simulink model "cx06_MA"  (Simulink 7.5)
settings: Solver=FixedStepDiscrete  StartTime=0.0  StopTime=10.0  RelTol=1e-3
undefined symbols (not defined in the file or in its folder): DiscIntNeverNeededParam, ECU555, int, motohawk_build_version, motohawk_trunc_name, motohawk_vardec_path
libraries: MotoHawk_lib x811, simulink x43, simulink_need_slupdate x1
(part 3 of 10)

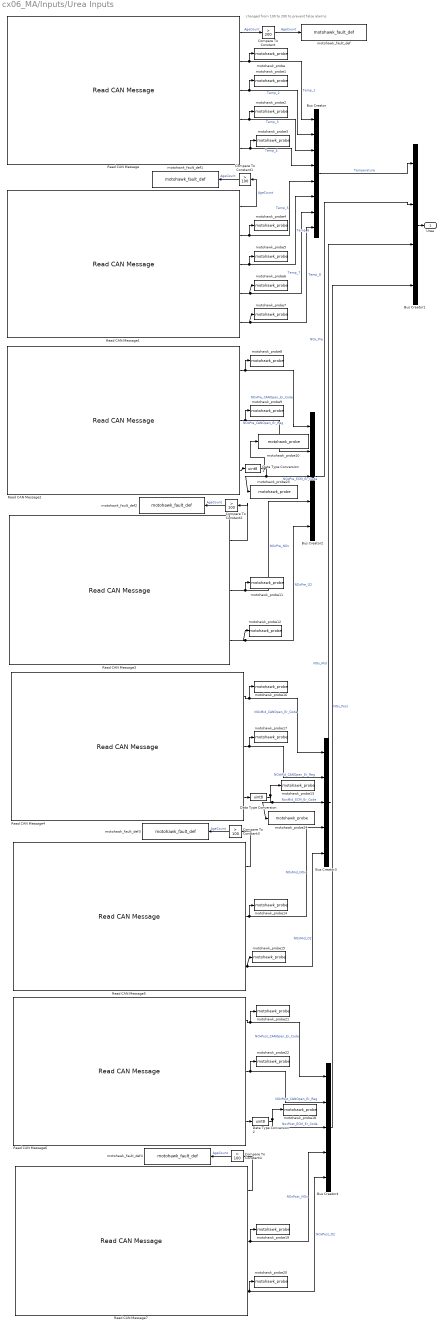
== system cx06_MA/Inputs/Urea Inputs ==
  note: changed from 100 to 200 to prevent false alarms
  Bus Creator : BusCreator  Inputs=8
  Bus Creator1 : BusCreator
  Bus Creator2 : BusCreator  Inputs=5
  Bus Creator3 : BusCreator  Inputs=5
  Bus Creator4 : BusCreator  Inputs=5
  Compare To Constant : simulink/Logic and Bit Operations/Compare To Constant  SystemSampleTime=-1  relop=>  const=200  LogicOutDataTypeMode=boolean  ZeroCross=off
  Compare To Constant{1..4} (4 alike) : simulink/Logic and Bit Operations/Compare To Constant  SystemSampleTime=-1  relop=>  const=100  LogicOutDataTypeMode=boolean  ZeroCross=off
  Data Type Conversion : DataTypeConversion  OutDataTypeMode=uint8  OutDataType=sfix(16)  OutScaling=2^0  OutDataTypeStr=uint8
  Data Type Conversion1 : DataTypeConversion  OutDataTypeMode=uint8  OutDataType=sfix(16)  OutScaling=2^0  OutDataTypeStr=uint8
  Data Type Conversion2 : DataTypeConversion  OutDataTypeMode=uint8  OutDataType=sfix(16)  OutScaling=2^0  OutDataTypeStr=uint8
  Read CAN Message : MotoHawk_lib/CAN Blocks/Read CAN Message  nam=['CAN_' num2str(1)]  bus=-2  msg=CANRx_Temp_1A4  queue=1  slot=''  valid=off  stale=on  labelwires=on
  Read CAN Message1 : MotoHawk_lib/CAN Blocks/Read CAN Message  nam=['CAN_' num2str(1)]  bus=-2  msg=CANRx_Temp_1A5  queue=1  slot=''  valid=off  stale=on  labelwires=on
  Read CAN Message2 : MotoHawk_lib/CAN Blocks/Read CAN Message  nam=['CAN_' num2str(1)]  bus=-2  msg=CANRx_NOx_A3  queue=1  slot=''  valid=off  stale=off  labelwires=off
  Read CAN Message3 : MotoHawk_lib/CAN Blocks/Read CAN Message  nam=['CAN_' num2str(1)]  bus=-2  msg=CANRx_NOx_1A3  queue=1  slot=''  valid=off  stale=on  labelwires=off
  Read CAN Message4 : MotoHawk_lib/CAN Blocks/Read CAN Message  nam=['CAN_' num2str(1)]  bus=-2  msg=CANRx_NOx_A1  queue=1  slot=''  valid=off  stale=off  labelwires=off
  Read CAN Message5 : MotoHawk_lib/CAN Blocks/Read CAN Message  nam=['CAN_' num2str(1)]  bus=-2  msg=CANRx_NOx_1A1  queue=1  slot=''  valid=off  stale=on  labelwires=off
  Read CAN Message6 : MotoHawk_lib/CAN Blocks/Read CAN Message  nam=['CAN_' num2str(1)]  bus=-2  msg=CANRx_NOx_A2  queue=1  slot=''  valid=off  stale=off  labelwires=off
  Read CAN Message7 : MotoHawk_lib/CAN Blocks/Read CAN Message  nam=['CAN_' num2str(1)]  bus=-2  msg=CANRx_NOx_1A2  queue=1  slot=''  valid=off  stale=on  labelwires=off
  motohawk_fault_def : MotoHawk_lib/Fault Management Blocks/motohawk_fault_def  nam='Temp1A4'  mode=Enabled - Persistent  id=[]  x=10  y=11  input_suspected=on  indeterminate=off  increment_xy=on  downsample_count=1  ovr_cals=on  ovr_actions=on  show_actions=on  action1_name='Urea_Inject'  action1_cond=Active  action2_name=''  action2_cond=(None)  action3_name=''  action3_cond=(None)  action4_name=''  action4_cond=(None)
  motohawk_fault_def1 : MotoHawk_lib/Fault Management Blocks/motohawk_fault_def  nam='Temp1A5'  mode=Enabled - Persistent  id=[]  x=10  y=11  input_suspected=on  indeterminate=off  increment_xy=on  downsample_count=1  ovr_cals=on  ovr_actions=on  show_actions=on  action1_name=''  action1_cond=(None)  action2_name=''  action2_cond=(None)  action3_name=''  action3_cond=(None)  action4_name=''  action4_cond=(None)
  motohawk_fault_def2 : MotoHawk_lib/Fault Management Blocks/motohawk_fault_def  nam='NOxPre_CAN'  mode=Enabled - Persistent  id=[]  x=10  y=11  input_suspected=on  indeterminate=off  increment_xy=on  downsample_count=1  ovr_cals=on  ovr_actions=on  show_actions=on  action1_name='Urea_Inject'  action1_cond=Active  action2_name=''  action2_cond=(None)  action3_name=''  action3_cond=(None)  action4_name=''  action4_cond=(None)
  motohawk_fault_def3 : MotoHawk_lib/Fault Management Blocks/motohawk_fault_def  nam='NOxMid_CAN'  mode=Enabled - Persistent  id=[]  x=10  y=11  input_suspected=on  indeterminate=off  increment_xy=on  downsample_count=1  ovr_cals=on  ovr_actions=on  show_actions=on  action1_name=''  action1_cond=(None)  action2_name=''  action2_cond=(None)  action3_name=''  action3_cond=(None)  action4_name=''  action4_cond=(None)
  motohawk_fault_def4 : MotoHawk_lib/Fault Management Blocks/motohawk_fault_def  nam='NOxPost_CAN'  mode=Enabled - Persistent  id=[]  x=10  y=11  input_suspected=on  indeterminate=off  increment_xy=on  downsample_count=1  ovr_cals=on  ovr_actions=on  show_actions=on  action1_name=''  action1_cond=(None)  action2_name=''  action2_cond=(None)  action3_name=''  action3_cond=(None)  action4_name=''  action4_cond=(None)
  motohawk_probe{,1..9,11..12,14..17,19..22} (20 alike) : MotoHawk_lib/Calibration & Probing Blocks/motohawk_probe  nam='Probe'  show_more=on  name_source=Use Input Wire Name  read_level=1  view_as=Number  enum_struct={'Disabled', 'Enabled'}  vector_style=Wide Row  use_help_units=off  help=''  units=''  use_header_enum=off  row_header_enum={}  col_header_enum={}  use_precision=off  precision=''  gain=1  offset=0  exp=1  use_mototune_group=off  mototune_group=motohawk_vardec_path(gcb)
  motohawk_probe10 : MotoHawk_lib/Calibration & Probing Blocks/motohawk_probe  nam='Probe'  show_more=on  name_source=Use Input Wire Name  read_level=1  view_as=Enumeration  enum_struct=struct('name', {'All OK', '16b ADC failed to init', '+Vsw shorted', 'Sensor Turned Off', 'HTR Open', 'HTR Shorted', '1wire bus Shorted', 'No 1wire bus', 'CRC16 Error', 'Invalid 1wire par', '+Vsw < 9 for 7s', '+Vsw > 30V', 'VS > 1.5/1.6V', 'RVS > 280/300', 'VHerr > 0.5V', 'VP1+ > 6V', 'VP2+ < 2V', 'VP2 out range', '.25V>VS+>.75V', 'UserData Corrupt', 'Invld SW State', 'CAN overrun', 'CAN passive', 'CAN heartbeat', 'CAN recover bus off', 'CAN TxID col', 'Serial Overrun'}, 'value', {0, 17, 18, 19, 20, 21, 33, 34, 35, 36, 49, 50, 65, 81, 82, 97, 98, 99, 100, 101, 161, 177, 178, 179, 180, 181, 182})  vector_style=Wide Row  use_help_units=off  help=''  units=''  use_header_enum=off  row_header_enum={}  col_header_enum={}  use_precision=off  precision=''  gain=1  offset=0  exp=1  use_mototune_group=off  mototune_group=motohawk_vardec_path(gcb)
  motohawk_probe13 : MotoHawk_lib/Calibration & Probing Blocks/motohawk_probe  nam='Probe'  show_more=on  name_source=Use Input Wire Name  read_level=1  view_as=Enumeration  enum_struct=struct('name', {'All OK', '16b ADC failed to init', '+Vsw shorted', 'Sensor Turned Off', 'HTR Open', 'HTR Shorted', '1wire bus Shorted', 'No 1wire bus', 'CRC16 Error', 'Invalid 1wire par', '+Vsw < 9 for 7s', '+Vsw > 30V', 'VS > 1.5/1.6V', 'RVS > 280/300', 'VHerr > 0.5V', 'VP1+ > 6V', 'VP2+ < 2V', 'VP2 out range', '.25V>VS+>.75V', 'UserData Corrupt', 'Invld SW State', 'CAN overrun', 'CAN passive', 'CAN heartbeat', 'CAN recover bus off', 'CAN TxID col', 'Serial Overrun'}, 'value', {0, 17, 18, 19, 20, 21, 33, 34, 35, 36, 49, 50, 65, 81, 82, 97, 98, 99, 100, 101, 161, 177, 178, 179, 180, 181, 182})  vector_style=Wide Row  use_help_units=off  help=''  units=''  use_header_enum=off  row_header_enum={}  col_header_enum={}  use_precision=off  precision=''  gain=1  offset=0  exp=1  use_mototune_group=off  mototune_group=motohawk_vardec_path(gcb)
  motohawk_probe18 : MotoHawk_lib/Calibration & Probing Blocks/motohawk_probe  nam='Probe'  show_more=on  name_source=Use Input Wire Name  read_level=1  view_as=Enumeration  enum_struct=struct('name', {'All OK', '16b ADC failed to init', '+Vsw shorted', 'Sensor Turned Off', 'HTR Open', 'HTR Shorted', '1wire bus Shorted', 'No 1wire bus', 'CRC16 Error', 'Invalid 1wire par', '+Vsw < 9 for 7s', '+Vsw > 30V', 'VS > 1.5/1.6V', 'RVS > 280/300', 'VHerr > 0.5V', 'VP1+ > 6V', 'VP2+ < 2V', 'VP2 out range', '.25V>VS+>.75V', 'UserData Corrupt', 'Invld SW State', 'CAN overrun', 'CAN passive', 'CAN heartbeat', 'CAN recover bus off', 'CAN TxID col', 'Serial Overrun'}, 'value', {0, 17, 18, 19, 20, 21, 33, 34, 35, 36, 49, 50, 65, 81, 82, 97, 98, 99, 100, 101, 161, 177, 178, 179, 180, 181, 182})  vector_style=Wide Row  use_help_units=off  help=''  units=''  use_header_enum=off  row_header_enum={}  col_header_enum={}  use_precision=off  precision=''  gain=1  offset=0  exp=1  use_mototune_group=off  mototune_group=motohawk_vardec_path(gcb)
  motohawk_probe23 : MotoHawk_lib/Calibration & Probing Blocks/motohawk_probe  nam='NOxPre_ECM_Er_Raw'  show_more=on  name_source=Use Parameter  read_level=1  view_as=Number  enum_struct={'Disabled', 'Enabled'}  vector_style=Wide Row  use_help_units=off  help=''  units=''  use_header_enum=off  row_header_enum={}  col_header_enum={}  use_precision=off  precision=''  gain=1  offset=0  exp=1  use_mototune_group=off  mototune_group=motohawk_vardec_path(gcb)
  motohawk_probe24 : MotoHawk_lib/Calibration & Probing Blocks/motohawk_probe  nam='NOxMid_ECM_Er_Raw'  show_more=on  name_source=Use Parameter  read_level=1  view_as=Number  enum_struct={'Disabled', 'Enabled'}  vector_style=Wide Row  use_help_units=off  help=''  units=''  use_header_enum=off  row_header_enum={}  col_header_enum={}  use_precision=off  precision=''  gain=1  offset=0  exp=1  use_mototune_group=off  mototune_group=motohawk_vardec_path(gcb)
  Urea : Outport  OutDataType=sfix(16)  OutScaling=2^0
  wires:
  Compare To Constant/1 -> motohawk_fault_def/1  "AgeCount"
  Read CAN Message/1 -> Compare To Constant/1  "AgeCount"
  Read CAN Message/2 -> Bus Creator/1, motohawk_probe/1  "Temp_1"
  Read CAN Message/3 -> Bus Creator/2, motohawk_probe1/1  "Temp_2"
  Read CAN Message/4 -> Bus Creator/3, motohawk_probe2/1  "Temp_3"
  Read CAN Message/5 -> Bus Creator/4, motohawk_probe3/1  "Temp_4"
  Compare To Constant1/1 -> motohawk_fault_def1/1  "AgeCount"
  Read CAN Message1/1 -> Compare To Constant1/1  "AgeCount"
  Read CAN Message1/2 -> Bus Creator/5, motohawk_probe4/1  "Temp_5"
  Read CAN Message1/3 -> Bus Creator/6, motohawk_probe5/1  "Temp_6"
  Read CAN Message1/4 -> Bus Creator/7, motohawk_probe6/1  "Temp_7"
  Read CAN Message1/5 -> Bus Creator/8, motohawk_probe7/1  "Temp_8"
  Bus Creator/1 -> Bus Creator1/1  "Temperature"
  Bus Creator1/1 -> Urea/1
  Read CAN Message2/1 -> Bus Creator2/1, motohawk_probe8/1  "NOxPre_CANOpen_Er_Code"
  Read CAN Message2/2 -> Bus Creator2/2, motohawk_probe9/1  "NOxPre_CANOpen_Er_Reg"
  Read CAN Message2/3 -> Data Type Conversion1/1
  Compare To Constant2/1 -> motohawk_fault_def2/1  "AgeCount"
  Read CAN Message3/1 -> Compare To Constant2/1
  Read CAN Message3/2 -> Bus Creator2/4, motohawk_probe11/1  "NOxPre_NOx"
  Read CAN Message3/3 -> Bus Creator2/5, motohawk_probe12/1  "NOxPre_O2"
  Bus Creator2/1 -> Bus Creator1/2  "NOx_Pre"
  Read CAN Message4/1 -> motohawk_probe16/1, Bus Creator3/1  "NOxMid_CANOpen_Er_Code"
  Read CAN Message4/2 -> motohawk_probe17/1, Bus Creator3/2  "NOxMid_CANOpen_Er_Reg"
  Read CAN Message4/3 -> Data Type Conversion/1
  Compare To Constant3/1 -> motohawk_fault_def3/1  "AgeCount"
  Read CAN Message5/1 -> Compare To Constant3/1
  Read CAN Message5/2 -> Bus Creator3/4, motohawk_probe14/1  "NOxMid_NOx"
  Read CAN Message5/3 -> Bus Creator3/5, motohawk_probe15/1  "NOxMid_O2"
  Bus Creator3/1 -> Bus Creator1/3  "NOx_Mid"
  Data Type Conversion/1 -> motohawk_probe13/1, Bus Creator3/3, motohawk_probe24/1  "NoxMid_ECM_Er_Code"
  Data Type Conversion1/1 -> motohawk_probe10/1, Bus Creator2/3, motohawk_probe23/1  "NOxPre_ECM_Er_Code"
  Read CAN Message6/1 -> Bus Creator4/1, motohawk_probe21/1  "NOxPost_CANOpen_Er_Code"
  Read CAN Message6/2 -> Bus Creator4/2, motohawk_probe22/1  "NOxPost_CANOpen_Er_Reg"
  Read CAN Message6/3 -> Data Type Conversion2/1
  Compare To Constant4/1 -> motohawk_fault_def4/1  "AgeCount"
  Read CAN Message7/1 -> Compare To Constant4/1
  Read CAN Message7/2 -> motohawk_probe19/1, Bus Creator4/4  "NOxPost_NOx"
  Read CAN Message7/3 -> motohawk_probe20/1, Bus Creator4/5  "NOxPost_O2"
  Data Type Conversion2/1 -> Bus Creator4/3, motohawk_probe18/1  "NoxPost_ECM_Er_Code"
  Bus Creator4/1 -> Bus Creator1/4  "NOx_Post"

== system cx06_MA/MainState/Call Startup Event ==
  Trigger : TriggerPort  TriggerType=falling
  Function-Call Generator : simulink/Ports & Subsystems/Function-Call Generator  sample_time=-1  numberOfIterations=1
  Post Shutdown two ticks before MPRD off : MotoHawk_lib/Trigger Blocks/motohawk_event_call  SystemSampleTime=-1  mode=Post Event  trigger=STARTUP_EVENT  target=ECU555_80
  motohawk_code_coverage : MotoHawk_lib/Extra Development Blocks/motohawk_code_coverage
  wires:
  Function-Call Generator/1 -> Post Shutdown two ticks before MPRD off/Trigger

== system cx06_MA/MainState/Post Shutdown two ticks before MPRD off ==
  Trigger : TriggerPort  TriggerType=falling
  Function-Call Generator : simulink/Ports & Subsystems/Function-Call Generator  sample_time=-1  numberOfIterations=1
  Post Shutdown two ticks before MPRD off : MotoHawk_lib/Trigger Blocks/motohawk_event_call  SystemSampleTime=-1  mode=Post Event  trigger=SHUTDOWN_EVENT  target=ECU555_80
  motohawk_code_coverage : MotoHawk_lib/Extra Development Blocks/motohawk_code_coverage
  wires:
  Function-Call Generator/1 -> Post Shutdown two ticks before MPRD off/Trigger

== system cx06_MA/MainState/Save NV Vars one tick before MPRD off ==
  Trigger : TriggerPort  TriggerType=falling
  Function-Call Generator : simulink/Ports & Subsystems/Function-Call Generator  sample_time=-1  numberOfIterations=1
  Save NV Vars one tick before MPRD off : MotoHawk_lib/Data Storage Blocks/motohawk_store_nvmem  SystemSampleTime=-1
  motohawk_code_coverage : MotoHawk_lib/Extra Development Blocks/motohawk_code_coverage
  wires:
  Function-Call Generator/1 -> Save NV Vars one tick before MPRD off/Trigger

== system cx06_MA/MainState/Shutdown power on ECU565-128 ==
  Trigger : TriggerPort  TriggerType=falling
  Function-Call Generator : simulink/Ports & Subsystems/Function-Call Generator  sample_time=-1  numberOfIterations=1
  Shutdown power on ECU565-128 : MotoHawk_lib/Extra Development Blocks/motohawk_shutdown_power  SystemSampleTime=-1
  motohawk_code_coverage : MotoHawk_lib/Extra Development Blocks/motohawk_code_coverage
  wires:
  Function-Call Generator/1 -> Shutdown power on ECU565-128/Trigger

== system cx06_MA/Outputs/ARDAQ Outputs ==
  In1 : Inport  OutDataType=sfix(16)  OutScaling=2^0
  Bus Selector1 : BusSelector  OutputSignals="JCI.Voltage,JCI.Current,JCI.SOC,Analog.Driver.Brake,Fiat.Engine Torque.Eng_Torq_Actual,Fiat.Engine  General Status.Fuel_Inj_Roll_Cnt"
  Constant : Constant  OutDataType=sfix(16)  OutScaling=2^0
  Constant{1..3,5} (4 alike) : Constant  Value=0  OutDataType=sfix(16)  OutScaling=2^0
  Gain : Gain  Gain=100  ParameterDataType=sfix(16)  ParameterScaling=2^0  OutDataType=sfix(16)  OutScaling=2^0
  Product : Product  OutDataType=sfix(16)  OutScaling=2^0  RndMeth=Zero
  Send CAN Messages : MotoHawk_lib/CAN Blocks/Send CAN Messages  bus=-2  nam=['CAN_' num2str(2)]  msgl=ARDAQ_cX_430  pace=100  labelwires=on
  Send CAN Messages1 : MotoHawk_lib/CAN Blocks/Send CAN Messages  bus=-2  nam=['CAN_' num2str(2)]  msgl=ARDAQ_cX_431  pace=100  labelwires=on
  Send CAN Messages2 : MotoHawk_lib/CAN Blocks/Send CAN Messages  bus=-2  nam=['CAN_' num2str(2)]  msgl=ARDAQ_cX_432  pace=100  labelwires=on
  motohawk_calibration : MotoHawk_lib/Calibration & Probing Blocks/motohawk_calibration  nam='H2_Tank_Pres_Cal'  val=69  storage=Calibration  show_more=on  name_source=Use Parameter  data_type=int8  read_level=1  write_level=1  ovr_cals=on  view_as=Number  enum_struct={'Disabled', 'Enabled'}  vector_style=Wide Row  use_help_units=off  help=''  units=''  use_header_enum=off  row_header_enum={}  col_header_enum={}  use_min_max=on  min_val=-inf  max_val=inf  use_precision=off  precision=''  gain=1  offset=0  exp=1  use_mototune_group=off  mototune_group=motohawk_vardec_path(gcb)
  motohawk_calibration4 : MotoHawk_lib/Calibration & Probing Blocks/motohawk_calibration  nam='Fuel_Consumption_Adjustment'  val=1  storage=Calibration  show_more=on  name_source=Use Parameter  data_type=Inherit from 'Default Value'  read_level=1  write_level=1  ovr_cals=on  view_as=Number  enum_struct={'Disabled', 'Enabled'}  vector_style=Wide Row  use_help_units=off  help=''  units=''  use_header_enum=off  row_header_enum={}  col_header_enum={}  use_min_max=on  min_val=0  max_val=1  use_precision=on  precision='1.4'  gain=1  offset=0  exp=1  use_mototune_group=off  mototune_group=motohawk_vardec_path(gcb)
  motohawk_override_abs : MotoHawk_lib/Calibration & Probing Blocks/motohawk_override_abs  SystemSampleTime=-1  parent_name='ARDAQ_Fuel_Used'  parent_val=0  show_more=off  name_source=Use Parameter  parent_read_level=1  parent_override_level=1  view_as=Number  enum_struct={'Disabled', 'Enabled'}  use_help_units=off  parent_help=''  parent_units=''  use_min_max=off  parent_min=-inf  parent_max=inf  use_precision=off  parent_precision=''  parent_gain=1  parent_offset=0  parent_exp=1  use_mototune_group=off  parent_group=motohawk_vardec_path(gcb)
  motohawk_override_abs1 : MotoHawk_lib/Calibration & Probing Blocks/motohawk_override_abs  SystemSampleTime=-1  parent_name='ARDAQ_Engine_Torque'  parent_val=0  show_more=off  name_source=Use Parameter  parent_read_level=1  parent_override_level=1  view_as=Number  enum_struct={'Disabled', 'Enabled'}  use_help_units=off  parent_help=''  parent_units=''  use_min_max=off  parent_min=-inf  parent_max=inf  use_precision=off  parent_precision=''  parent_gain=1  parent_offset=0  parent_exp=1  use_mototune_group=off  parent_group=motohawk_vardec_path(gcb)
  wires:
  Constant/1 -> Send CAN Messages/7  "Fuel_B20"
  Constant3/1 -> Send CAN Messages/6  "Fuel_RFG"
  Constant1/1 -> Send CAN Messages/8  "Fuel_H2"
  Constant2/1 -> Send CAN Messages/5  "Fuel_E85"
  In1/1 -> Bus Selector1/1
  Bus Selector1/1 -> Send CAN Messages/1  "<Voltage>"
  Bus Selector1/2 -> Send CAN Messages/2  "<Current>"
  Bus Selector1/3 -> Send CAN Messages/3  "<SOC>"
  motohawk_calibration/1 -> Send CAN Messages1/1  "H2_Tank_Pres"
  Constant5/1 -> Send CAN Messages1/2  "H2_Tank_Temp"
  Bus Selector1/5 -> motohawk_override_abs1/1  "<Eng_Torq_Actual>"
  Bus Selector1/4 -> Gain/1  "<Brake>"
  Gain/1 -> Send CAN Messages/4  "Brake_Pedal_Pos"
  motohawk_override_abs/1 -> Send CAN Messages1/3  "Liquid_Fuel_Used"
  motohawk_override_abs1/1 -> Send CAN Messages2/1  "EngTrq"
  motohawk_calibration4/1 -> Product/2
  Bus Selector1/6 -> Product/1  "<Fuel_Inj_Roll_Cnt>"
  Product/1 -> motohawk_override_abs/1  "Liquid_Fuel_Used"

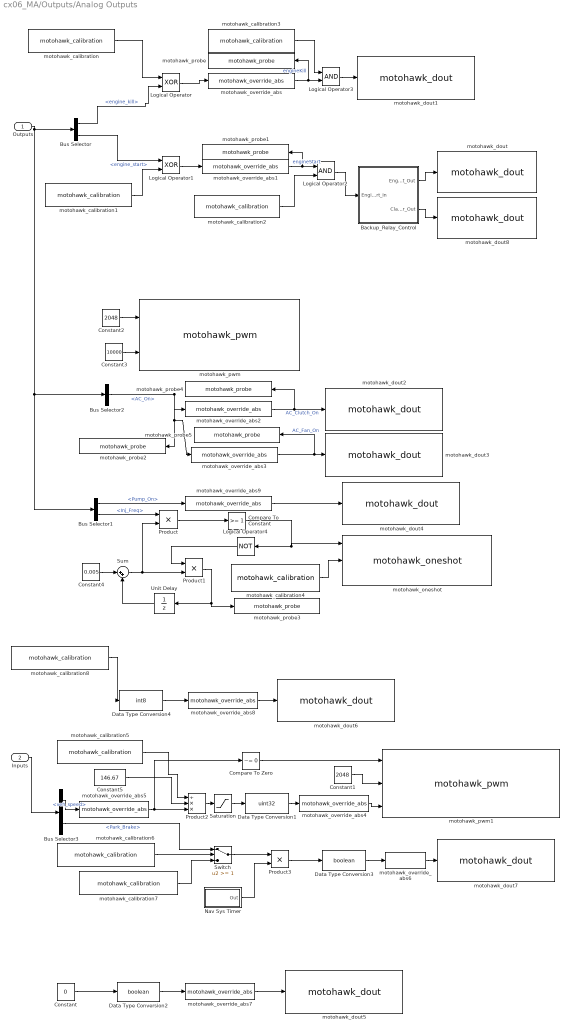
== system cx06_MA/Outputs/Analog Outputs ==
  Outputs : Inport  OutDataType=sfix(16)  OutScaling=2^0
  Inputs : Inport  Port=2  OutDataType=sfix(16)  OutScaling=2^0
  Backup_Relay_Control : Subsystem
  Bus Selector : BusSelector  OutputSignals=Hybrid.engine_kill,Hybrid.engine_start
  Bus Selector1 : BusSelector  OutputSignals=Urea.Pump_On,Urea.Inj_Freq
  Bus Selector2 : BusSelector  OutputSignals=AC.AC_On
  Bus Selector3 : BusSelector  OutputSignals=IPT.Status 2.veh_speed,GMLAN.Park_Brake
  Compare To Constant : simulink/Logic and Bit Operations/Compare To Constant  SystemSampleTime=-1  relop=>=  const=1  LogicOutDataTypeMode=boolean  ZeroCross=off
  Compare To Zero : simulink/Logic and Bit Operations/Compare To Zero  SystemSampleTime=-1  relop=~=  LogicOutDataTypeMode=boolean  ZeroCross=off
  Constant : Constant  Value=0  OutDataType=fixdt(1, 16)  OutScaling=2^0
  Constant1 : Constant  Value=2048  OutDataTypeMode=int16  OutDataType=sfix(16)  OutScaling=2^0  OutDataTypeStr=int16
  Constant2 : Constant  Value=2048  OutDataType=sfix(16)  OutScaling=2^0  OutDataTypeStr=Inherit: Inherit via back propagation
  Constant3 : Constant  Value=10000  OutDataType=sfix(16)  OutScaling=2^0  OutDataTypeStr=Inherit: Inherit via back propagation
  Constant4 : Constant  Value=0.005  OutDataType=sfix(16)  OutScaling=2^0
  Constant5 : Constant  Value=146.67  OutDataType=sfix(16)  OutScaling=2^0
  Data Type Conversion1 : DataTypeConversion  OutDataTypeMode=uint32  OutDataType=sfix(16)  OutScaling=2^0  OutDataTypeStr=uint32
  Data Type Conversion2 : DataTypeConversion  OutDataTypeMode=boolean  OutDataType=sfix(16)  OutScaling=2^0  OutDataTypeStr=boolean
  Data Type Conversion3 : DataTypeConversion  OutDataTypeMode=boolean  OutDataType=sfix(16)  OutScaling=2^0  OutDataTypeStr=boolean
  Data Type Conversion4 : DataTypeConversion  OutDataTypeMode=int8  OutDataType=sfix(16)  OutScaling=2^0  OutDataTypeStr=int8
  Logical Operator : Logic  Operator=XOR  AllPortsSameDT=off  OutDataTypeMode=boolean  OutDataTypeStr=boolean
  Logical Operator1 : Logic  Operator=XOR  AllPortsSameDT=off  OutDataTypeMode=boolean  LogicDataType=uint(16)  OutDataTypeStr=boolean
  Logical Operator2 : Logic  AllPortsSameDT=off  OutDataTypeMode=boolean  OutDataTypeStr=boolean
  Logical Operator3 : Logic  AllPortsSameDT=off  OutDataTypeMode=boolean  OutDataTypeStr=boolean
  Logical Operator4 : Logic  Operator=NOT  AllPortsSameDT=off  OutDataTypeMode=boolean  OutDataTypeStr=boolean
  Nav Sys Timer : Subsystem
  Product : Product  OutDataType=sfix(16)  OutScaling=2^0  RndMeth=Zero
  Product1 : Product  OutDataTypeMode=double  OutDataType=sfix(16)  OutScaling=2^0  OutDataTypeStr=double  RndMeth=Zero
  Product2 : Product  Inputs=/**  OutDataTypeMode=double  OutDataType=sfix(16)  OutScaling=2^0  OutDataTypeStr=double  RndMeth=Zero
  Product3 : Product  OutDataType=sfix(16)  OutScaling=2^0  RndMeth=Zero
  Saturation : Saturate  UpperLimit=inf  LowerLimit=2
  Sum : Sum  Inputs=|++  OutDataType=sfix(16)  OutScaling=2^0
  Switch : Switch  Threshold=1  ZeroCross=off
  Unit Delay : UnitDelay  SampleTime=-1
  motohawk_calibration : MotoHawk_lib/Calibration & Probing Blocks/motohawk_calibration  nam='EngineKill_Invert'  val=0  storage=Calibration  show_more=on  name_source=Use Parameter  data_type=uint8  read_level=1  write_level=1  ovr_cals=on  view_as=Number  enum_struct={'False', 'True'}  vector_style=Wide Row  use_help_units=on  help='Invert the output'  units=''  use_header_enum=off  row_header_enum={}  col_header_enum={}  use_min_max=off  min_val=-inf  max_val=inf  use_precision=off  precision=''  gain=1  offset=0  exp=1  use_mototune_group=off  mototune_group=motohawk_vardec_path(gcb)
  motohawk_calibration1 : MotoHawk_lib/Calibration & Probing Blocks/motohawk_calibration  nam='EngineStart_Invert'  val=0  storage=Calibration  show_more=on  name_source=Use Parameter  data_type=uint8  read_level=1  write_level=1  ovr_cals=on  view_as=Number  enum_struct={'False', 'True'}  vector_style=Wide Row  use_help_units=on  help='Invert the Output'  units=''  use_header_enum=off  row_header_enum={}  col_header_enum={}  use_min_max=off  min_val=-inf  max_val=inf  use_precision=off  precision=''  gain=1  offset=0  exp=1  use_mototune_group=off  mototune_group=motohawk_vardec_path(gcb)
  motohawk_calibration2 : MotoHawk_lib/Calibration & Probing Blocks/motohawk_calibration  nam='EngineStart_Enable'  val=1  storage=Calibration  show_more=on  name_source=Use Parameter  data_type=uint8  read_level=1  write_level=1  ovr_cals=on  view_as=Number  enum_struct={'False', 'True'}  vector_style=Wide Row  use_help_units=on  help='Invert the Output'  units=''  use_header_enum=off  row_header_enum={}  col_header_enum={}  use_min_max=off  min_val=-inf  max_val=inf  use_precision=off  precision=''  gain=1  offset=0  exp=1  use_mototune_group=off  mototune_group=motohawk_vardec_path(gcb)
  motohawk_calibration3 : MotoHawk_lib/Calibration & Probing Blocks/motohawk_calibration  nam='EngineKill_Enable'  val=1  storage=Calibration  show_more=on  name_source=Use Parameter  data_type=uint8  read_level=1  write_level=1  ovr_cals=on  view_as=Number  enum_struct={'False', 'True'}  vector_style=Wide Row  use_help_units=on  help='Invert the output'  units=''  use_header_enum=off  row_header_enum={}  col_header_enum={}  use_min_max=off  min_val=-inf  max_val=inf  use_precision=off  precision=''  gain=1  offset=0  exp=1  use_mototune_group=off  mototune_group=motohawk_vardec_path(gcb)
  motohawk_calibration4 : MotoHawk_lib/Calibration & Probing Blocks/motohawk_calibration  nam='Urea_PulseW'  val=5000  storage=Calibration  show_more=on  name_source=Use Parameter  data_type=int32  read_level=1  write_level=1  ovr_cals=on  view_as=Number  enum_struct={'False', 'True'}  vector_style=Wide Row  use_help_units=on  help='Length of time the injector is on'  units='ms'  use_header_enum=off  row_header_enum={}  col_header_enum={}  use_min_max=off  min_val=-inf  max_val=inf  use_precision=on  precision='1.2'  gain=0.001  offset=0  exp=1  use_mototune_group=off  mototune_group=motohawk_vardec_path(gcb)
  motohawk_calibration5 : MotoHawk_lib/Calibration & Probing Blocks/motohawk_calibration  nam='Nav_Ft_per_Pulse'  val=1  storage=Calibration  show_more=on  name_source=Use Parameter  data_type=single  read_level=1  write_level=1  ovr_cals=on  view_as=Number  enum_struct={'Disabled', 'Enabled'}  vector_style=Wide Row  use_help_units=off  help=''  units=''  use_header_enum=off  row_header_enum={}  col_header_enum={}  use_min_max=on  min_val=0.1  max_val=inf  use_precision=off  precision=''  gain=1  offset=0  exp=1  use_mototune_group=off  mototune_group=motohawk_vardec_path(gcb)
  motohawk_calibration6 : MotoHawk_lib/Calibration & Probing Blocks/motohawk_calibration  nam='Nav_DVD_Safety'  val=0  storage=Calibration  show_more=on  name_source=Use Parameter  data_type=int8  read_level=1  write_level=1  ovr_cals=on  view_as=Enumeration  enum_struct={'Disabled', 'Enabled'}  vector_style=Wide Row  use_help_units=off  help=''  units=''  use_header_enum=off  row_header_enum={}  col_header_enum={}  use_min_max=on  min_val=0  max_val=inf  use_precision=off  precision=''  gain=1  offset=0  exp=1  use_mototune_group=off  mototune_group=motohawk_vardec_path(gcb)
  motohawk_calibration7 : MotoHawk_lib/Calibration & Probing Blocks/motohawk_calibration  nam='Nav_DVD_Unsafe_Value'  val=1  storage=Calibration  show_more=on  name_source=Use Parameter  data_type=int8  read_level=1  write_level=1  ovr_cals=on  view_as=Number  enum_struct={'Disabled', 'Enabled'}  vector_style=Wide Row  use_help_units=off  help=''  units=''  use_header_enum=off  row_header_enum={}  col_header_enum={}  use_min_max=on  min_val=-10  max_val=inf  use_precision=off  precision=''  gain=1  offset=0  exp=1  use_mototune_group=off  mototune_group=motohawk_vardec_path(gcb)
  motohawk_calibration8 : MotoHawk_lib/Calibration & Probing Blocks/motohawk_calibration  nam='Batt_Fan_Circuit'  val=0  storage=Calibration  show_more=on  name_source=Use Parameter  data_type=int8  read_level=1  write_level=1  ovr_cals=on  view_as=Number  enum_struct={'Disabled', 'Enabled'}  vector_style=Wide Row  use_help_units=off  help=''  units=''  use_header_enum=off  row_header_enum={}  col_header_enum={}  use_min_max=on  min_val=-10  max_val=inf  use_precision=off  precision=''  gain=1  offset=0  exp=1  use_mototune_group=off  mototune_group=motohawk_vardec_path(gcb)
  motohawk_dout : MotoHawk_lib/Digital I//O Blocks/motohawk_dout  text_resource=FINJ1  code_resource=NONE  val_resource=-1  target=ECU555-80  resource_enum_str=(None)=-1,FUELP=0,HSOL1=2,HSOL2=3,HSOL3=4,HSOL4=5,START=6,OILP=11,FINJ1=12,FINJ2=13,FINJ3=14,FINJ4=15,FINJ5=16,FINJ6=17,AINJ1=18,AINJ2=19,AINJ3=20,AINJ4=21,AINJ5=22,AINJ6=23,TACH=24,EST 1=36,EST 2=37,EST 3=38,EST 4=39,EST 5=40,EST 6=41,EST 7=42,EST 8=43,MPRD=52  use_diag=off  use_vardec=off  nam='EngineStart_Pin'  read_level=1  write_level=1  group='I/O Pins | Outputs Config'
  motohawk_dout1 : MotoHawk_lib/Digital I//O Blocks/motohawk_dout  text_resource=FINJ2  code_resource=NONE  val_resource=-1  target=ECU555-80  resource_enum_str=(None)=-1,FUELP=0,HSOL1=2,HSOL2=3,HSOL3=4,HSOL4=5,START=6,OILP=11,FINJ1=12,FINJ2=13,FINJ3=14,FINJ4=15,FINJ5=16,FINJ6=17,AINJ1=18,AINJ2=19,AINJ3=20,AINJ4=21,AINJ5=22,AINJ6=23,TACH=24,EST 1=36,EST 2=37,EST 3=38,EST 4=39,EST 5=40,EST 6=41,EST 7=42,EST 8=43,MPRD=52  use_diag=off  use_vardec=off  nam='EngineKill_Pin'  read_level=1  write_level=1  group='I/O Pins | Outputs Config'
  motohawk_dout2 : MotoHawk_lib/Digital I//O Blocks/motohawk_dout  text_resource=FINJ4  code_resource=NONE  val_resource=-1  target=ECU555-80  resource_enum_str=(None)=-1,FUELP=0,HSOL1=2,HSOL2=3,HSOL3=4,HSOL4=5,START=6,OILP=11,FINJ1=12,FINJ2=13,FINJ3=14,FINJ4=15,FINJ5=16,FINJ6=17,AINJ1=18,AINJ2=19,AINJ3=20,AINJ4=21,AINJ5=22,AINJ6=23,TACH=24,EST 1=36,EST 2=37,EST 3=38,EST 4=39,EST 5=40,EST 6=41,EST 7=42,EST 8=43,MPRD=52  use_diag=off  use_vardec=on  nam='AC_Clutch'  read_level=1  write_level=1  group='I/O Pins | Outputs Config'
  motohawk_dout3 : MotoHawk_lib/Digital I//O Blocks/motohawk_dout  text_resource=AINJ3  code_resource=NONE  val_resource=-1  target=ECU555-80  resource_enum_str=(None)=-1,FUELP=0,HSOL1=2,HSOL2=3,HSOL3=4,HSOL4=5,START=6,OILP=11,FINJ1=12,FINJ2=13,FINJ3=14,FINJ4=15,FINJ5=16,FINJ6=17,AINJ1=18,AINJ2=19,AINJ3=20,AINJ4=21,AINJ5=22,AINJ6=23,TACH=24,EST 1=36,EST 2=37,EST 3=38,EST 4=39,EST 5=40,EST 6=41,EST 7=42,EST 8=43,MPRD=52  use_diag=off  use_vardec=on  nam='AC_Fan'  read_level=1  write_level=1  group='I/O Pins | Outputs Config'
  motohawk_dout4 : MotoHawk_lib/Digital I//O Blocks/motohawk_dout  text_resource=AINJ1  code_resource=NONE  val_resource=-1  target=ECU555-80  resource_enum_str=(None)=-1,FUELP=0,HSOL1=2,HSOL2=3,HSOL3=4,HSOL4=5,START=6,OILP=11,FINJ1=12,FINJ2=13,FINJ3=14,FINJ4=15,FINJ5=16,FINJ6=17,AINJ1=18,AINJ2=19,AINJ3=20,AINJ4=21,AINJ5=22,AINJ6=23,TACH=24,EST 1=36,EST 2=37,EST 3=38,EST 4=39,EST 5=40,EST 6=41,EST 7=42,EST 8=43,MPRD=52  use_diag=off  use_vardec=on  nam='Urea_Power'  read_level=1  write_level=1  group='I/O Pins | Outputs Config'
  motohawk_dout5 : MotoHawk_lib/Digital I//O Blocks/motohawk_dout  text_resource=FINJ3  code_resource=NONE  val_resource=-1  target=ECU555-80  resource_enum_str=(None)=-1,FUELP=0,HSOL1=2,HSOL2=3,HSOL3=4,HSOL4=5,START=6,OILP=11,FINJ1=12,FINJ2=13,FINJ3=14,FINJ4=15,FINJ5=16,FINJ6=17,AINJ1=18,AINJ2=19,AINJ3=20,AINJ4=21,AINJ5=22,AINJ6=23,TACH=24,EST 1=36,EST 2=37,EST 3=38,EST 4=39,EST 5=40,EST 6=41,EST 7=42,EST 8=43,MPRD=52  use_diag=off  use_vardec=off  nam='AC_Fan'  read_level=1  write_level=1  group='I/O Pins | Outputs Config'
  motohawk_dout6 : MotoHawk_lib/Digital I//O Blocks/motohawk_dout  text_resource=AINJ4  code_resource=NONE  val_resource=-1  target=ECU555-80  resource_enum_str=(None)=-1,FUELP=0,HSOL1=2,HSOL2=3,HSOL3=4,HSOL4=5,START=6,OILP=11,FINJ1=12,FINJ2=13,FINJ3=14,FINJ4=15,FINJ5=16,FINJ6=17,AINJ1=18,AINJ2=19,AINJ3=20,AINJ4=21,AINJ5=22,AINJ6=23,TACH=24,EST 1=36,EST 2=37,EST 3=38,EST 4=39,EST 5=40,EST 6=41,EST 7=42,EST 8=43,MPRD=52  use_diag=off  use_vardec=off  nam='AC_Fan'  read_level=1  write_level=1  group='I/O Pins | Outputs Config'
  motohawk_dout7 : MotoHawk_lib/Digital I//O Blocks/motohawk_dout  text_resource=FINJ6  code_resource=NONE  val_resource=-1  target=ECU555-80  resource_enum_str=(None)=-1,FUELP=0,HSOL1=2,HSOL2=3,HSOL3=4,HSOL4=5,START=6,OILP=11,FINJ1=12,FINJ2=13,FINJ3=14,FINJ4=15,FINJ5=16,FINJ6=17,AINJ1=18,AINJ2=19,AINJ3=20,AINJ4=21,AINJ5=22,AINJ6=23,TACH=24,EST 1=36,EST 2=37,EST 3=38,EST 4=39,EST 5=40,EST 6=41,EST 7=42,EST 8=43,MPRD=52  use_diag=off  use_vardec=off  nam='AC_Fan'  read_level=1  write_level=1  group='I/O Pins | Outputs Config'
  motohawk_dout8 : MotoHawk_lib/Digital I//O Blocks/motohawk_dout  text_resource=AINJ2  code_resource=NONE  val_resource=-1  target=ECU555-80  resource_enum_str=(None)=-1,FUELP=0,HSOL1=2,HSOL2=3,HSOL3=4,HSOL4=5,START=6,OILP=11,FINJ1=12,FINJ2=13,FINJ3=14,FINJ4=15,FINJ5=16,FINJ6=17,AINJ1=18,AINJ2=19,AINJ3=20,AINJ4=21,AINJ5=22,AINJ6=23,TACH=24,EST 1=36,EST 2=37,EST 3=38,EST 4=39,EST 5=40,EST 6=41,EST 7=42,EST 8=43,MPRD=52  use_diag=off  use_vardec=off  nam='EngineStart_Pin'  read_level=1  write_level=1  group='I/O Pins | Outputs Config'
  motohawk_oneshot : MotoHawk_lib/Advanced Digital I//O/motohawk_oneshot  res_nam=[]  text_resource=HSOL1  code_resource=NONE  val_resource=-1  target=ECU555-80  resource_enum_str=(None)=-1,HSOL1=2,HSOL2=3,HSOL3=4,HSOL4=5,START=6,OILP=11,ESC=35,EST 1=36,EST 2=37,EST 3=38,EST 4=39,EST 5=40,EST 6=41,EST 7=42,EST 8=43  show_ports=on  use_vardec=on  nam='Urea_Injector'  read_level=1  write_level=1  group='I/O Pins | Outputs Config'
  motohawk_override_abs{,1..3} (4 alike) : MotoHawk_lib/Calibration & Probing Blocks/motohawk_override_abs  SystemSampleTime=-1  parent_name='Override_Absolute'  parent_val=0  show_more=on  name_source=Use Output Wire Name  parent_read_level=1  parent_override_level=1  view_as=Number  enum_struct={'Disabled', 'Enabled'}  use_help_units=off  parent_help=''  parent_units=''  use_min_max=off  parent_min=-inf  parent_max=inf  use_precision=off  parent_precision=''  parent_gain=1  parent_offset=0  parent_exp=1  use_mototune_group=off  parent_group=motohawk_vardec_path(gcb)
  motohawk_override_abs4 : MotoHawk_lib/Calibration & Probing Blocks/motohawk_override_abs  SystemSampleTime=-1  parent_name='Nav_Spd_Freq_100'  parent_val=200  show_more=on  name_source=Use Parameter  parent_read_level=1  parent_override_level=1  view_as=Number  enum_struct={'Disabled', 'Enabled'}  use_help_units=off  parent_help=''  parent_units=''  use_min_max=on  parent_min=-inf  parent_max=inf  use_precision=off  parent_precision=''  parent_gain=1  parent_offset=0  parent_exp=1  use_mototune_group=off  parent_group=motohawk_vardec_path(gcb)
  motohawk_override_abs5 : MotoHawk_lib/Calibration & Probing Blocks/motohawk_override_abs  SystemSampleTime=-1  parent_name='Nav_Veh_Spd'  parent_val=0  show_more=on  name_source=Use Parameter  parent_read_level=1  parent_override_level=1  view_as=Number  enum_struct={'Disabled', 'Enabled'}  use_help_units=off  parent_help=''  parent_units=''  use_min_max=on  parent_min=-inf  parent_max=inf  use_precision=off  parent_precision=''  parent_gain=1  parent_offset=0  parent_exp=1  use_mototune_group=off  parent_group=motohawk_vardec_path(gcb)
  motohawk_override_abs6 : MotoHawk_lib/Calibration & Probing Blocks/motohawk_override_abs  SystemSampleTime=-1  parent_name='Nav_Park'  parent_val=0  show_more=off  name_source=Use Parameter  parent_read_level=1  parent_override_level=1  view_as=Number  enum_struct={'Disabled', 'Enabled'}  use_help_units=off  parent_help=''  parent_units=''  use_min_max=off  parent_min=-inf  parent_max=inf  use_precision=off  parent_precision=''  parent_gain=1  parent_offset=0  parent_exp=1  use_mototune_group=off  parent_group=motohawk_vardec_path(gcb)
  motohawk_override_abs7 : MotoHawk_lib/Calibration & Probing Blocks/motohawk_override_abs  SystemSampleTime=-1  parent_name='ISO_Fault_LED'  parent_val=0  show_more=off  name_source=Use Parameter  parent_read_level=1  parent_override_level=1  view_as=Number  enum_struct={'Disabled', 'Enabled'}  use_help_units=off  parent_help=''  parent_units=''  use_min_max=off  parent_min=-inf  parent_max=inf  use_precision=off  parent_precision=''  parent_gain=1  parent_offset=0  parent_exp=1  use_mototune_group=off  parent_group=motohawk_vardec_path(gcb)
  motohawk_override_abs8 : MotoHawk_lib/Calibration & Probing Blocks/motohawk_override_abs  SystemSampleTime=-1  parent_name='Batt_Fan_Relay'  parent_val=0  show_more=on  name_source=Use Parameter  parent_read_level=1  parent_override_level=1  view_as=Number  enum_struct={'Disabled', 'Enabled'}  use_help_units=off  parent_help=''  parent_units=''  use_min_max=off  parent_min=-inf  parent_max=inf  use_precision=off  parent_precision=''  parent_gain=1  parent_offset=0  parent_exp=1  use_mototune_group=off  parent_group=motohawk_vardec_path(gcb)
  motohawk_override_abs9 : MotoHawk_lib/Calibration & Probing Blocks/motohawk_override_abs  SystemSampleTime=-1  parent_name='Urea_Pump_On'  parent_val=0  show_more=on  name_source=Use Parameter  parent_read_level=1  parent_override_level=1  view_as=Number  enum_struct={'Disabled', 'Enabled'}  use_help_units=off  parent_help=''  parent_units=''  use_min_max=off  parent_min=-inf  parent_max=inf  use_precision=off  parent_precision=''  parent_gain=1  parent_offset=0  parent_exp=1  use_mototune_group=off  parent_group=motohawk_vardec_path(gcb)
  motohawk_probe{,1..2,4..5} (5 alike) : MotoHawk_lib/Calibration & Probing Blocks/motohawk_probe  nam='Probe'  show_more=on  name_source=Use Input Wire Name  read_level=1  view_as=Number  enum_struct={'Disabled', 'Enabled'}  vector_style=Wide Row  use_help_units=off  help=''  units=''  use_header_enum=off  row_header_enum={}  col_header_enum={}  use_precision=off  precision=''  gain=1  offset=0  exp=1  use_mototune_group=off  mototune_group=motohawk_vardec_path(gcb)
  motohawk_probe3 : MotoHawk_lib/Calibration & Probing Blocks/motohawk_probe  nam='UreaTimeSinceInj'  show_more=off  name_source=Use Parameter  read_level=1  view_as=Number  enum_struct={'Disabled', 'Enabled'}  vector_style=Wide Row  use_help_units=off  help=''  units=''  use_header_enum=off  row_header_enum={}  col_header_enum={}  use_precision=off  precision=''  gain=1  offset=0  exp=1  use_mototune_group=off  mototune_group=motohawk_vardec_path(gcb)
  motohawk_pwm : MotoHawk_lib/Analog I//O Blocks/motohawk_pwm  res_name=[]  text_resource=ETC  code_resource=NONE  val_resource=-1  target=ECU555-80  resource_enum_str=(None)=-1,FUELP=0,ETC=1,HSOL1=2,HSOL2=3,HSOL3=4,HSOL4=5,START=6,OILP=11,FINJ1=12,FINJ2=13,FINJ3=14,FINJ4=15,FINJ5=16,FINJ6=17,AINJ1=18,AINJ2=19,AINJ3=20,AINJ4=21,AINJ5=22,AINJ6=23,TACH=24,EST 1=36,EST 2=37,EST 3=38,EST 4=39,EST 5=40,EST 6=41,EST 7=42,EST 8=43  freq_mode=-1  min_freq=2  use_max_freq=off  max_freq=42949672.96  use_enable=off  use_brake=off  output_current=off  output_fault_status=off  use_child=off  use_vardec=on  nam='IPT_EPO'  read_level=1  write_level=1  group='I/O Pins | Outputs Config'
  motohawk_pwm1 : MotoHawk_lib/Analog I//O Blocks/motohawk_pwm  res_name=[]  text_resource=EST 6  code_resource=NONE  val_resource=-1  target=ECU555-80  resource_enum_str=(None)=-1,FUELP=0,ETC=1,HSOL1=2,HSOL2=3,HSOL3=4,HSOL4=5,START=6,OILP=11,FINJ1=12,FINJ2=13,FINJ3=14,FINJ4=15,FINJ5=16,FINJ6=17,AINJ1=18,AINJ2=19,AINJ3=20,AINJ4=21,AINJ5=22,AINJ6=23,TACH=24,EST 1=36,EST 2=37,EST 3=38,EST 4=39,EST 5=40,EST 6=41,EST 7=42,EST 8=43  freq_mode=-1  min_freq=1  use_max_freq=off  max_freq=42949672.96  use_enable=on  use_brake=off  output_current=off  output_fault_status=off  use_child=off  use_vardec=off  nam='PWM'  read_level=1  write_level=1  group='System | I/O Pins | Outputs Config'
  wires:
  Outputs/1 -> Bus Selector/1, Bus Selector2/1, Bus Selector1/1
  Logical Operator/1 -> motohawk_override_abs/1
  Logical Operator1/1 -> motohawk_override_abs1/1
  motohawk_calibration/1 -> Logical Operator/1
  Bus Selector/2 -> Logical Operator1/1  "<engine_start>"
  motohawk_calibration1/1 -> Logical Operator1/2
  Bus Selector2/1 -> motohawk_probe2/1, motohawk_override_abs3/1, motohawk_override_abs2/1  "<AC_On>"
  Constant2/1 -> motohawk_pwm/1
  motohawk_override_abs/1 -> motohawk_probe/1, Logical Operator3/2  "engineKill"
  motohawk_override_abs1/1 -> motohawk_probe1/1, Logical Operator2/1  "engineStart"
  motohawk_calibration2/1 -> Logical Operator2/2
  motohawk_calibration3/1 -> Logical Operator3/1
  Logical Operator3/1 -> motohawk_dout1/1
  Unit Delay/1 -> Sum/2
  Constant4/1 -> Sum/1
  Product/1 -> Compare To Constant/1
  Compare To Constant/1 -> motohawk_oneshot/1, Logical Operator4/1
  Sum/1 -> Product1/2, Product/2
  Product1/1 -> Unit Delay/1, motohawk_probe3/1
  Logical Operator4/1 -> Product1/1
  motohawk_calibration4/1 -> motohawk_oneshot/2
  Bus Selector1/2 -> Product/1  "<Inj_Freq>"
  Bus Selector1/1 -> motohawk_override_abs9/1  "<Pump_On>"
  motohawk_override_abs2/1 -> motohawk_dout2/1, motohawk_probe4/1  "AC_Clutch_On"
  motohawk_override_abs3/1 -> motohawk_dout3/1, motohawk_probe5/1  "AC_Fan_On"
  Inputs/1 -> Bus Selector3/1
  Constant5/1 -> Product2/2
  Bus Selector3/1 -> motohawk_override_abs5/1  "<veh_speed>"
  motohawk_calibration5/1 -> Product2/1
  Data Type Conversion1/1 -> motohawk_override_abs4/1
  motohawk_calibration6/1 -> Switch/2
  Bus Selector3/2 -> Switch/1  "<Park_Brake>"
  motohawk_calibration7/1 -> Switch/3
  Data Type Conversion3/1 -> motohawk_override_abs6/1
  motohawk_override_abs6/1 -> motohawk_dout7/1
  Product2/1 -> Saturation/1
  Saturation/1 -> Data Type Conversion1/1
  motohawk_override_abs5/1 -> Product2/3, Compare To Zero/1
  Constant1/1 -> motohawk_pwm1/2
  motohawk_override_abs4/1 -> motohawk_pwm1/3
  Compare To Zero/1 -> motohawk_pwm1/1
  motohawk_override_abs7/1 -> motohawk_dout5/1
  Constant3/1 -> motohawk_pwm/2
  motohawk_override_abs8/1 -> motohawk_dout6/1
  Data Type Conversion2/1 -> motohawk_override_abs7/1
  Data Type Conversion4/1 -> motohawk_override_abs8/1
  Logical Operator2/1 -> Backup_Relay_Control/1(Engine_Start_In)
  Backup_Relay_Control/1(Engine_Start_Out) -> motohawk_dout/1
  Backup_Relay_Control/2(Clarion_Pwr_Out) -> motohawk_dout8/1
  Product3/1 -> Data Type Conversion3/1
  Switch/1 -> Product3/1
  Nav Sys Timer/1(Out) -> Product3/2
  Bus Selector/1 -> Logical Operator/2  "<engine_kill>"
  motohawk_override_abs9/1 -> motohawk_dout4/1
  Constant/1 -> Data Type Conversion2/1
  motohawk_calibration8/1 -> Data Type Conversion4/1

== system cx06_MA/Outputs/Debug Outputs ==
  note: Hybrid State
      | 0 - Safety
      | 1 - Diesel
      | 2 - Regen
      | 3 - HEV
      | 4 - ZEV
  Outputs : Inport  OutDataType=sfix(16)  OutScaling=2^0
  In1 : Inport  Port=2  OutDataType=sfix(16)  OutScaling=2^0
  Bus Selector : BusSelector  OutputSignals=Hybrid.hybrid_state,Hybrid.TC_Outputs.front_slip,Hybrid.TC_Outputs.rear_slip,Hybrid.TC_Outputs.TC_Active
  Bus Selector1 : BusSelector  OutputSignals=Analog.Driver.Accel,Analog.Driver.Brake,Analog.Driver.Clutch,Analog.Trans.Neutral,Analog.Trans.Reverse
  Data Type Conversion{,1..5} (6 alike) : DataTypeConversion  OutDataTypeMode=uint8  OutDataType=sfix(16)  OutScaling=2^0  OutDataTypeStr=uint8  RndMeth=Nearest
  Gain : Gain  Gain=100  ParameterDataType=sfix(16)  ParameterScaling=2^0  OutDataType=sfix(16)  OutScaling=2^0
  Gain1 : Gain  Gain=100  ParameterDataType=sfix(16)  ParameterScaling=2^0  OutDataType=sfix(16)  OutScaling=2^0
  Gain2 : Gain  Gain=100  ParameterDataType=sfix(16)  ParameterScaling=2^0  OutDataType=sfix(16)  OutScaling=2^0
  Send CAN Messages : MotoHawk_lib/CAN Blocks/Send CAN Messages  bus=-2  nam=['CAN_' num2str(1)]  msgl=CANTx_DEBUG_350  pace=500  labelwires=on
  wires:
  Outputs/1 -> Bus Selector/1
  In1/1 -> Bus Selector1/1
  Gain/1 -> Send CAN Messages/2  "Accel"
  Gain2/1 -> Send CAN Messages/1  "Brake"
  Gain1/1 -> Send CAN Messages/4  "Clutch"
  Bus Selector1/1 -> Gain/1  "<Accel>"
  Bus Selector1/2 -> Gain2/1  "<Brake>"
  Bus Selector1/3 -> Gain1/1  "<Clutch>"
  Data Type Conversion/1 -> Send CAN Messages/5  "Neutral"
  Bus Selector1/4 -> Data Type Conversion/1  "<Neutral>"
  Data Type Conversion1/1 -> Send CAN Messages/6  "Reverse"
  Bus Selector1/5 -> Data Type Conversion1/1  "<Reverse>"
  Data Type Conversion2/1 -> Send CAN Messages/3  "HEV_State"
  Bus Selector/1 -> Data Type Conversion2/1  "<hybrid_state>"
  Bus Selector/3 -> Data Type Conversion3/1  "<rear_slip>"
  Data Type Conversion3/1 -> Send CAN Messages/7  "Front_Slip?"
  Bus Selector/2 -> Data Type Conversion4/1  "<front_slip>"
  Data Type Conversion4/1 -> Send CAN Messages/8  "Rear_Slip?"
  Bus Selector/4 -> Data Type Conversion5/1  "<TC_Active>"
  Data Type Conversion5/1 -> Send CAN Messages/9  "TC_Active"
